simulink library "PhaseCheck"  (Simulink 8.8)
settings: Solver=ode45  StartTime=0.0  StopTime=10.0  RelTol=1e-3  EnableMultiTasking=on
libraries: carnot x1
settings Model: Creator=lena.frank  LastModifiedBy=User

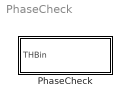
== system PhaseCheck ==
  PhaseCheck : Subsystem  mask(phasecheck){}
      mask help: Checks whether fluid is still in the correct phase, for example if water is not steam or ice. Simulation is stopped for inconstistent phase.
      mask Help: web(fullfile(path_carnot('help'),'phase_check.html'),'-helpbrowser')

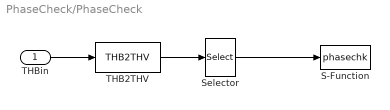
== system PhaseCheck/PhaseCheck ==
  THBin : Inport
  S-Function : S-Function  FunctionName=phasechk  SFunctionDeploymentMode=off  EnableBusSupport=off
  Selector : Selector  InputPortWidth=20  IndexOptions=Index vector (dialog)  Indices=[2:6]  OutputSizes=1
  THB2THV : carnot/Toolbox/THB2THV
  wires:
  THB2THV/1 -> Selector/1
  THBin/1 -> THB2THV/1
  Selector/1 -> S-Function/1
